simulink library "csu_tfl_thruster_forces_lander_lib"  (R2014b)
settings: Solver=ode45  StartTime=0.0  StopTime=10.0  RelTol=1e-3
libraries: util_thruster_lib x25, util_info_lib x1
settings Model: Creator=Nilesh  LastModifiedBy=mstewart

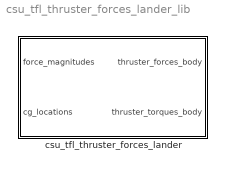
== system csu_tfl_thruster_forces_lander_lib ==
  csu_tfl_thruster_forces_lander : Subsystem

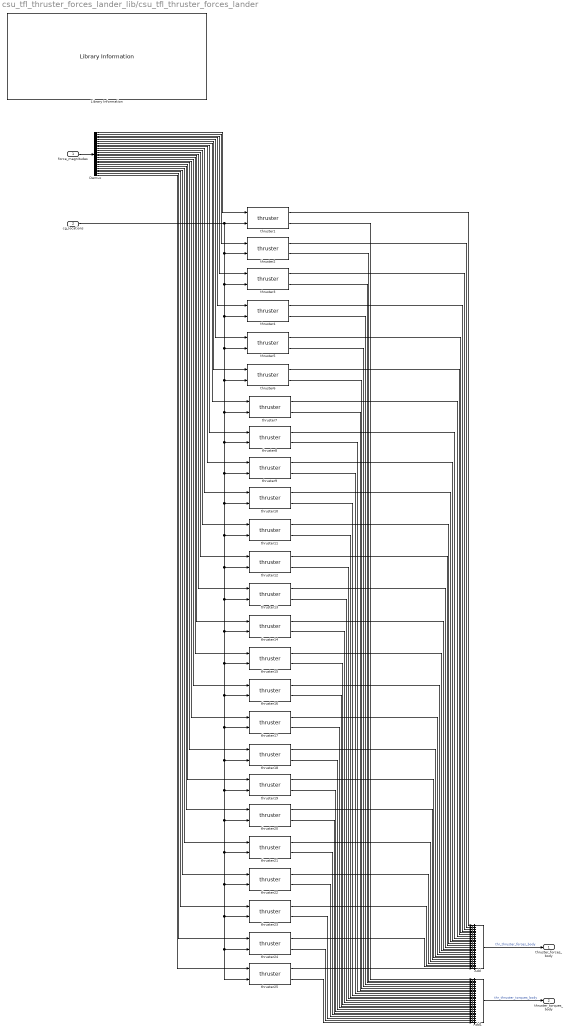
== system csu_tfl_thruster_forces_lander_lib/csu_tfl_thruster_forces_lander ==
  force_magnitudes : Inport
  cg_locations : Inport  Port=2
  Add : Sum  Inputs=+++++++++++++++++++++++++
  Add1 : Sum  Inputs=+++++++++++++++++++++++++
  Demux : Demux  Outputs=25
  Library Information : util_info_lib/Library Information  owner='NONE'
  thruster1 : util_thruster_lib/thruster  Thruster_Position=tfl_thruster1_position  Thruster_Orientation=tfl_thruster1_orientation
  thruster10 : util_thruster_lib/thruster  Thruster_Position=tfl_thruster10_position  Thruster_Orientation=tfl_thruster10_orientation
  thruster11 : util_thruster_lib/thruster  Thruster_Position=tfl_thruster11_position  Thruster_Orientation=tfl_thruster11_orientation
  thruster12 : util_thruster_lib/thruster  Thruster_Position=tfl_thruster12_position  Thruster_Orientation=tfl_thruster12_orientation
  thruster13 : util_thruster_lib/thruster  Thruster_Position=tfl_thruster13_position  Thruster_Orientation=tfl_thruster13_orientation
  thruster14 : util_thruster_lib/thruster  Thruster_Position=tfl_thruster14_position  Thruster_Orientation=tfl_thruster14_orientation
  thruster15 : util_thruster_lib/thruster  Thruster_Position=tfl_thruster15_position  Thruster_Orientation=tfl_thruster15_orientation
  thruster16 : util_thruster_lib/thruster  Thruster_Position=tfl_thruster16_position  Thruster_Orientation=tfl_thruster16_orientation
  thruster17 : util_thruster_lib/thruster  Thruster_Position=tfl_thruster17_position  Thruster_Orientation=tfl_thruster17_orientation
  thruster18 : util_thruster_lib/thruster  Thruster_Position=tfl_thruster18_position  Thruster_Orientation=tfl_thruster18_orientation
  thruster19 : util_thruster_lib/thruster  Thruster_Position=tfl_thruster19_position  Thruster_Orientation=tfl_thruster19_orientation
  thruster2 : util_thruster_lib/thruster  Thruster_Position=tfl_thruster2_position  Thruster_Orientation=tfl_thruster2_orientation
  thruster20 : util_thruster_lib/thruster  Thruster_Position=tfl_thruster20_position  Thruster_Orientation=tfl_thruster20_orientation
  thruster21 : util_thruster_lib/thruster  Thruster_Position=tfl_thruster21_position  Thruster_Orientation=tfl_thruster21_orientation
  thruster22 : util_thruster_lib/thruster  Thruster_Position=tfl_thruster22_position  Thruster_Orientation=tfl_thruster22_orientation
  thruster23 : util_thruster_lib/thruster  Thruster_Position=tfl_thruster23_position  Thruster_Orientation=tfl_thruster23_orientation
  thruster24 : util_thruster_lib/thruster  Thruster_Position=tfl_thruster24_position  Thruster_Orientation=tfl_thruster24_orientation
  thruster25 : util_thruster_lib/thruster  Thruster_Position=tfl_thruster25_position  Thruster_Orientation=tfl_thruster25_orientation
  thruster3 : util_thruster_lib/thruster  Thruster_Position=tfl_thruster3_position  Thruster_Orientation=tfl_thruster3_orientation
  thruster4 : util_thruster_lib/thruster  Thruster_Position=tfl_thruster4_position  Thruster_Orientation=tfl_thruster4_orientation
  thruster5 : util_thruster_lib/thruster  Thruster_Position=tfl_thruster5_position  Thruster_Orientation=tfl_thruster5_orientation
  thruster6 : util_thruster_lib/thruster  Thruster_Position=tfl_thruster6_position  Thruster_Orientation=tfl_thruster6_orientation
  thruster7 : util_thruster_lib/thruster  Thruster_Position=tfl_thruster7_position  Thruster_Orientation=tfl_thruster7_orientation
  thruster8 : util_thruster_lib/thruster  Thruster_Position=tfl_thruster8_position  Thruster_Orientation=tfl_thruster8_orientation
  thruster9 : util_thruster_lib/thruster  Thruster_Position=tfl_thruster9_position  Thruster_Orientation=tfl_thruster9_orientation
  thruster_forces_body : Outport
  thruster_torques_body : Outport  Port=2
  wires:
  cg_locations/1 -> thruster7/2, thruster16/2, thruster18/2, thruster19/2, thruster23/2, thruster25/2, thruster24/2, thruster22/2, thruster21/2, thruster20/2, thruster17/2, thruster15/2, thruster14/2, thruster13/2, thruster12/2, thruster11/2, thruster10/2, thruster9/2, thruster8/2, thruster6/2, thruster5/2, thruster4/2, thruster3/2, thruster2/2, thruster1/2
  force_magnitudes/1 -> Demux/1
  Add1/1 -> thruster_torques_body/1  "thr_thruster_torques_body"
  thruster1/1 -> Add/1
  thruster2/1 -> Add/2
  thruster3/1 -> Add/3
  Demux/1 -> thruster1/1
  Demux/2 -> thruster2/1
  Demux/3 -> thruster3/1
  Demux/4 -> thruster4/1
  Demux/5 -> thruster5/1
  Demux/6 -> thruster6/1
  Demux/7 -> thruster7/1
  thruster1/2 -> Add1/1
  thruster2/2 -> Add1/2
  thruster3/2 -> Add1/3
  thruster4/2 -> Add1/4
  thruster5/2 -> Add1/5
  thruster6/2 -> Add1/6
  thruster7/2 -> Add1/7
  Add/1 -> thruster_forces_body/1  "thr_thruster_forces_body"
  Demux/8 -> thruster8/1
  Demux/9 -> thruster9/1
  Demux/10 -> thruster10/1
  Demux/11 -> thruster11/1
  Demux/12 -> thruster12/1
  Demux/13 -> thruster13/1
  Demux/14 -> thruster14/1
  Demux/15 -> thruster15/1
  Demux/16 -> thruster16/1
  Demux/17 -> thruster17/1
  Demux/18 -> thruster18/1
  Demux/19 -> thruster19/1
  Demux/20 -> thruster20/1
  Demux/21 -> thruster21/1
  Demux/22 -> thruster22/1
  Demux/23 -> thruster23/1
  Demux/24 -> thruster24/1
  Demux/25 -> thruster25/1
  thruster4/1 -> Add/4
  thruster5/1 -> Add/5
  thruster6/1 -> Add/6
  thruster7/1 -> Add/7
  thruster8/1 -> Add/8
  thruster9/1 -> Add/9
  thruster10/1 -> Add/10
  thruster11/1 -> Add/11
  thruster12/1 -> Add/12
  thruster13/1 -> Add/13
  thruster14/1 -> Add/14
  thruster15/1 -> Add/15
  thruster16/1 -> Add/16
  thruster17/1 -> Add/17
  thruster18/1 -> Add/18
  thruster19/1 -> Add/19
  thruster20/1 -> Add/20
  thruster21/1 -> Add/21
  thruster22/1 -> Add/22
  thruster23/1 -> Add/23
  thruster24/1 -> Add/24
  thruster25/1 -> Add/25
  thruster8/2 -> Add1/8
  thruster9/2 -> Add1/9
  thruster10/2 -> Add1/10
  thruster11/2 -> Add1/11
  thruster12/2 -> Add1/12
  thruster13/2 -> Add1/13
  thruster14/2 -> Add1/14
  thruster15/2 -> Add1/15
  thruster16/2 -> Add1/16
  thruster17/2 -> Add1/17
  thruster18/2 -> Add1/18
  thruster19/2 -> Add1/19
  thruster20/2 -> Add1/20
  thruster21/2 -> Add1/21
  thruster22/2 -> Add1/22
  thruster23/2 -> Add1/23
  thruster24/2 -> Add1/24
  thruster25/2 -> Add1/25
